simulink model "MODEL"  (R2016b)
settings: Solver=FixedStepAuto  StartTime=0.0  StopTime=30  FixedStep=0.001  RelTol=1e-3
values from neighbouring files (symbols this model uses):
  b = 0.1    [Input_LQR.m]    (also in main.m)
  g = 9.81    [Input_LQR.m]    (also in main.m)
  k = 0.15    [Input_LQR.m]    (also in main.m)
  L = 1.4    [Input_LQR.m]    (also in main.m = 0.9)
  M = 1    [Input_LQR.m]    (also in main.m)
  m = 3/4    (= 0.75)    [Input_LQR.m]    (also in main.m)
  theta_0 = 0    [Input_LQR.m]    (also in main.m = 1.57079632679)
  theta_dot0 = 0    [Input_LQR.m]    (also in main.m)
  x_0 = 0    [Input_LQR.m]    (also in main.m)
  x_dot0 = 0    [Input_LQR.m]    (also in main.m)
settings Model: Creator=sbuadu  LastModifiedBy=sbuadu

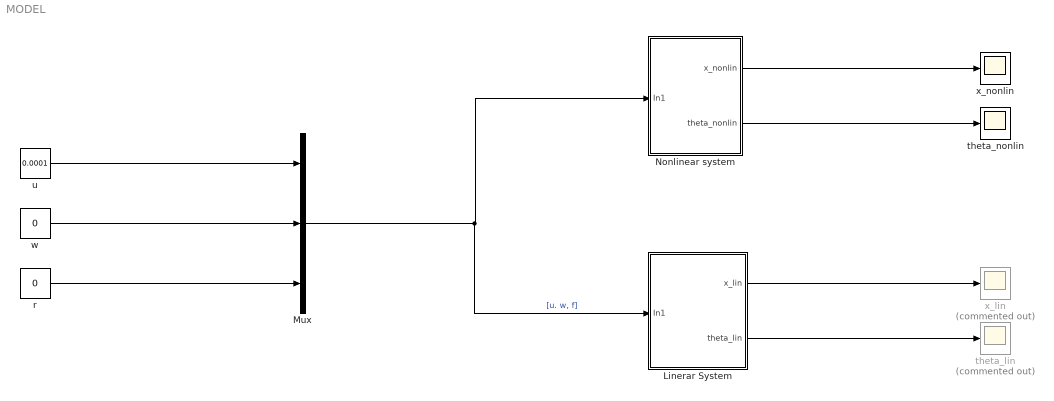
== system MODEL ==
  Linerar System : Subsystem
  Mux : Mux  Inputs=3
  "Nonlinear system " : Subsystem
  r : Constant  Value=0  SampleTime=0.01
  theta_lin : Scope  Commented=on
  "theta_nonlin " : Scope
  u : Constant  Value=0.0001  VectorParams1D=off  SampleTime=0.01
  w : Constant  Value=0  SampleTime=0.01
  x_lin : Scope  Commented=on
  x_nonlin : Scope
  wires:
  r/1 -> Mux/3
  w/1 -> Mux/2
  Mux/1 -> Linerar System/1(In1), "Nonlinear system "/1(In1)  "[u. w, f]"
  "Nonlinear system "/1(x_nonlin) -> x_nonlin/1
  "Nonlinear system "/2(theta_nonlin) -> "theta_nonlin "/1
  u/1 -> Mux/1
  Linerar System/1(x_lin) -> x_lin/1
  Linerar System/2(theta_lin) -> theta_lin/1

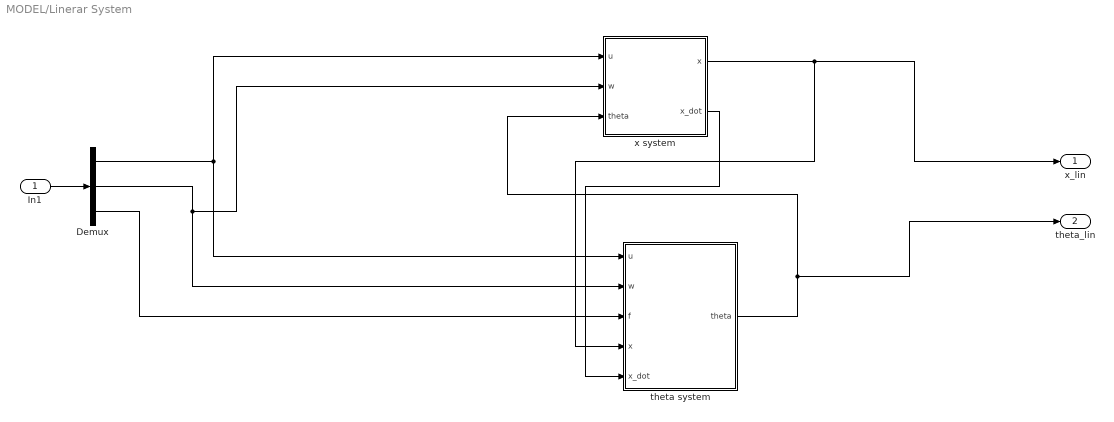
== system MODEL/Linerar System ==
  In1 : Inport
  Demux : Demux  Outputs=3
  "theta system " : Subsystem
  x system : Subsystem
  x_lin : Outport
  theta_lin : Outport  Port=2
  wires:
  x system/1(x) -> "theta system "/4(x), x_lin/1
  Demux/2 -> "theta system "/2(w), x system/2(w)
  "theta system "/1(theta) -> theta_lin/1, x system/3(theta)
  Demux/3 -> "theta system "/3(f)
  x system/2(x_dot) -> "theta system "/5(x_dot)
  In1/1 -> Demux/1
  Demux/1 -> x system/1("u "), "theta system "/1("u ")

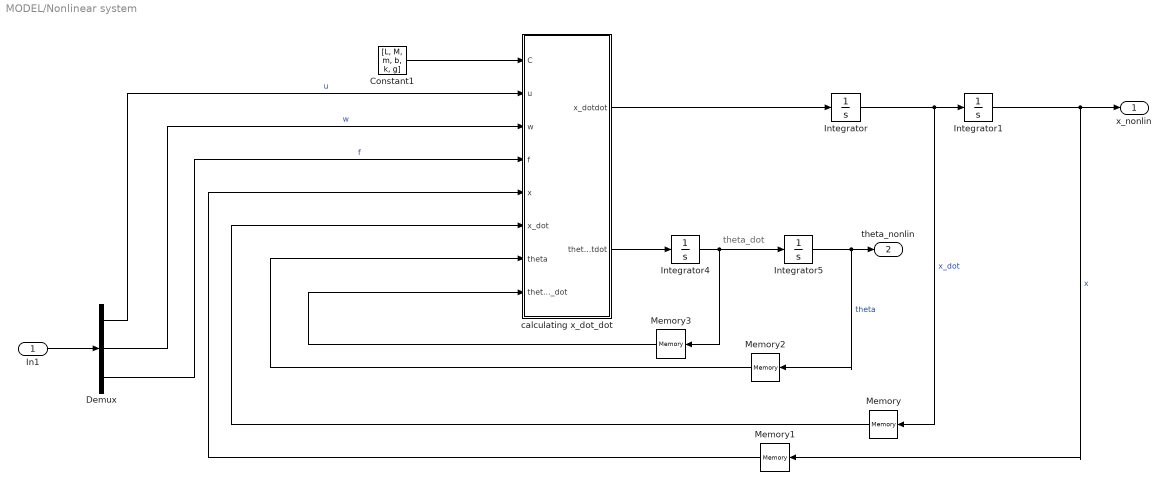
== system MODEL/Nonlinear system  ==
  note: theta_dot
  In1 : Inport
  Constant1 : Constant  Value=[L, M, m, b, k, g]  SampleTime=0.01
  Demux : Demux  Outputs=3
  Integrator{,1,4..5} (4 alike) : Integrator
  Memory : Memory  X0=x_dot0
  Memory1 : Memory  X0=x_0
  Memory2 : Memory  X0=theta_0
  Memory3 : Memory  X0=theta_dot0
  calculating x_dot_dot : MATLAB Function  TreatAsAtomicUnit=on
  x_nonlin : Outport
  theta_nonlin : Outport  Port=2
  wires:
  In1/1 -> Demux/1
  Demux/1 -> calculating x_dot_dot/2(u)  "u"
  Demux/2 -> calculating x_dot_dot/3(w)  "w"
  Demux/3 -> calculating x_dot_dot/4(f)  "f"
  calculating x_dot_dot/1(x_dotdot) -> Integrator/1
  Integrator/1 -> Memory/1, Integrator1/1  "x_dot"
  Integrator1/1 -> Memory1/1, x_nonlin/1  "x"
  Constant1/1 -> calculating x_dot_dot/1(C)
  calculating x_dot_dot/2(theta_dotdot) -> Integrator4/1
  Integrator4/1 -> Memory3/1, Integrator5/1
  Integrator5/1 -> Memory2/1, theta_nonlin/1  "theta"
  Memory1/1 -> calculating x_dot_dot/5(x)
  Memory/1 -> calculating x_dot_dot/6(x_dot)
  Memory2/1 -> calculating x_dot_dot/7(theta)
  Memory3/1 -> calculating x_dot_dot/8(theta_dot)

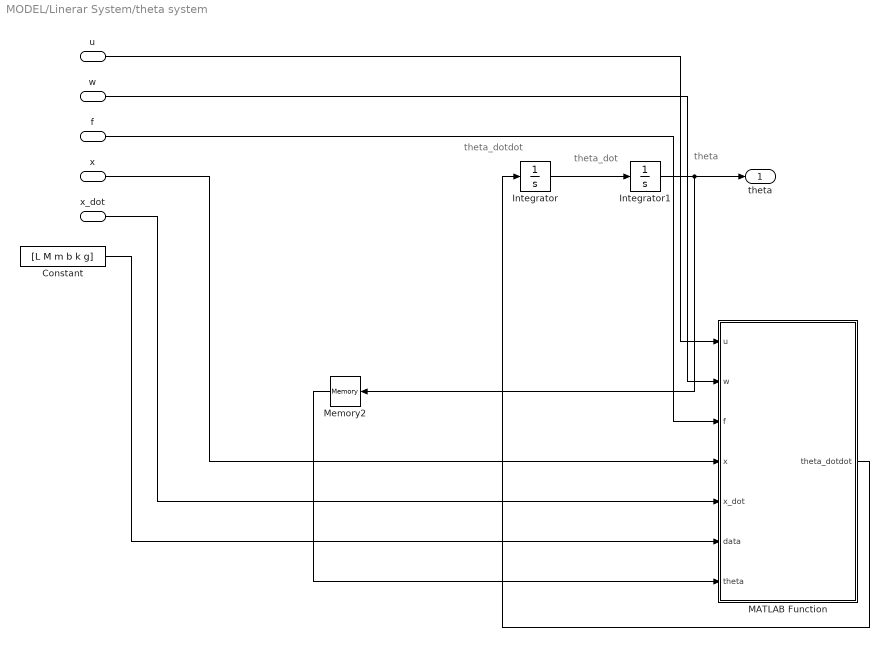
== system MODEL/Linerar System/theta system  ==
  note: theta
  note: theta_dotdot
  note: theta_dot
  "u " : Inport
  w : Inport  Port=2
  f : Inport  Port=3
  x : Inport  Port=4
  x_dot : Inport  Port=5
  Constant : Constant  Value=[L M m b k g]  VectorParams1D=off  SampleTime=0.01
  Integrator : Integrator  InitialCondition=theta_dot0
  Integrator1 : Integrator  InitialCondition=theta_0
  MATLAB Function : MATLAB Function  TreatAsAtomicUnit=on
  Memory2 : Memory  X0=theta_0
  theta : Outport
  wires:
  MATLAB Function/1(theta_dotdot) -> Integrator/1
  Integrator/1 -> Integrator1/1
  "u "/1 -> MATLAB Function/1(u)
  w/1 -> MATLAB Function/2(w)
  x/1 -> MATLAB Function/4(x)
  Integrator1/1 -> Memory2/1, theta/1
  Constant/1 -> MATLAB Function/6(data)
  f/1 -> MATLAB Function/3(f)
  x_dot/1 -> MATLAB Function/5(x_dot)
  Memory2/1 -> MATLAB Function/7(theta)

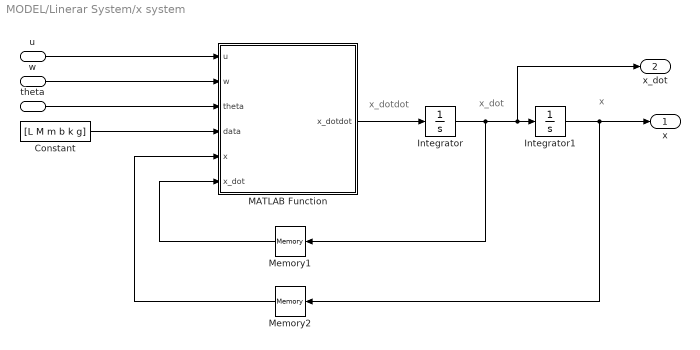
== system MODEL/Linerar System/x system ==
  note: x
  note: x_dotdot
  note: x_dot
  "u " : Inport
  w : Inport  Port=2
  theta : Inport  Port=3
  Constant : Constant  Value=[L M m b k g]  VectorParams1D=off  SampleTime=0.01
  Integrator : Integrator  InitialCondition=x_dot0
  Integrator1 : Integrator  InitialCondition=x_0
  MATLAB Function : MATLAB Function  TreatAsAtomicUnit=on
  Memory1 : Memory  X0=x_dot0
  Memory2 : Memory  X0=x_0
  x : Outport
  x_dot : Outport  Port=2
  wires:
  MATLAB Function/1(x_dotdot) -> Integrator/1
  Memory1/1 -> MATLAB Function/6(x_dot)
  Integrator/1 -> x_dot/1, Integrator1/1, Memory1/1
  "u "/1 -> MATLAB Function/1(u)
  w/1 -> MATLAB Function/2(w)
  theta/1 -> MATLAB Function/3(theta)
  Integrator1/1 -> Memory2/1, x/1
  Memory2/1 -> MATLAB Function/5(x)
  Constant/1 -> MATLAB Function/4(data)

== matlab function MODEL/Linerar System/x system/MATLAB Function ==
  data: u input; w input; theta input; data input; x_dotdot output; x input; x_dot input
function x_dotdot  = fcn(u,w,theta,data,x,x_dot)
L=data(1);
M=data(2);
m=data(3);
b=data(4);
k=data(5);
g=data(6);

x_dotdot=(u-w-m*g*theta*180/pi-b*x_dot-k*x)/(M);


end

== matlab function MODEL/Nonlinear system /calculating x_dot_dot ==
  data: C input; u input; x_dotdot output; w input; f input; x input; x_dot input; theta input; theta_dot input; theta_dotdot output
function [x_dotdot, theta_dotdot]= fcn(C,u, w, f, x, x_dot, theta, theta_dot)
%extracting the know parameters from vector C
L = C(1); 
M= C(2); 
m=C(3); 
b = C(4); 
k = C(5); 
g = C(6);

%calculating x_dot_dot
 x_dotdot = (u - f - w + f*cos(theta)^2 ...
            + m*L*theta_dot^2*sin(theta) ...
            -m*g*sin(theta)*cos(theta)...
            -b*x_dot -k*x )/(M + m*sin(theta)^2); 

%calculating theta_dot_dot
 theta_dotdot = (-u*cos(theta)+w*cos(theta)...
                   -M*L*theta_dot^2*sin(theta)*cos(theta)...
                    +(m+M)*g*sin(theta)-(M/m)*f*cos(theta)...
                    +b*x_dot*cos(theta)...
                    + k*x*cos(theta))/(L*(M+m*sin(theta)^2));

== matlab function MODEL/Linerar System/theta system /MATLAB Function ==
  data: u input; w input; f input; x input; x_dot input; data input; theta input; theta_dotdot output
function theta_dotdot  = fcn(u,w,f,x,x_dot,data,theta)
L=data(1);
M=data(2);
m=data(3);
b=data(4);
k=data(5);
g=data(6);

theta_dotdot=(-u+w+(m+M)*g*theta-(M/m)*f+b*x_dot+k*x)/(L*M);

end
